simulink model "send_udp"  (R2016a)
settings: Solver=FixedStepAuto  StartTime=0.0  StopTime=inf  RelTol=1e-3
libraries: simulink_extras x4, etargetslib x2, instrumentlib x1
settings Model: Creator=Florian Wachter  LastModifiedBy=Florian Wachter

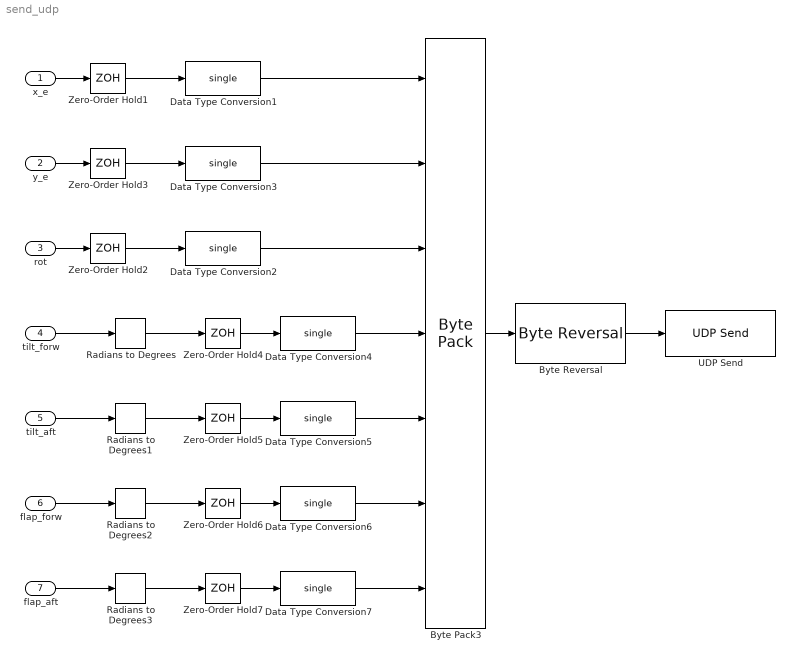
== system send_udp ==
  x_e : Inport
  y_e : Inport  Port=2
  rot : Inport  Port=3
  tilt_forw : Inport  Port=4
  tilt_aft : Inport  Port=5
  flap_forw : Inport  Port=6
  flap_aft : Inport  Port=7
  Byte Pack3 : etargetslib/Byte Pack  datatypes={'single','single','single','single','single','single','single'}  byteAlign=1
  Byte Reversal : etargetslib/Byte Reversal  numInp=1
  Data Type Conversion{1..7} (7 alike) : DataTypeConversion  OutDataTypeStr=single
  Radians to Degrees{,1..3} (4 alike) : simulink_extras/Transformations/Radians to Degrees
  UDP Send : instrumentlib/UDP Send  Host=localhost  Port=25000  LocalPort=-1  EnableBlockingMode=off  ByteOrder=BigEndian
  Zero-Order Hold{1..7} (7 alike) : ZeroOrderHold  SampleTime=1/30
  wires:
  tilt_forw/1 -> Radians to Degrees/1
  flap_forw/1 -> Radians to Degrees2/1
  Zero-Order Hold1/1 -> Data Type Conversion1/1
  Zero-Order Hold4/1 -> Data Type Conversion4/1
  Zero-Order Hold5/1 -> Data Type Conversion5/1
  Data Type Conversion5/1 -> Byte Pack3/5
  Data Type Conversion6/1 -> Byte Pack3/6
  Zero-Order Hold6/1 -> Data Type Conversion6/1
  Data Type Conversion4/1 -> Byte Pack3/4
  Data Type Conversion1/1 -> Byte Pack3/1
  x_e/1 -> Zero-Order Hold1/1
  Zero-Order Hold3/1 -> Data Type Conversion3/1
  y_e/1 -> Zero-Order Hold3/1
  tilt_aft/1 -> Radians to Degrees1/1
  Byte Reversal/1 -> UDP Send/1
  Byte Pack3/1 -> Byte Reversal/1
  Zero-Order Hold2/1 -> Data Type Conversion2/1
  rot/1 -> Zero-Order Hold2/1
  Data Type Conversion3/1 -> Byte Pack3/2
  Data Type Conversion2/1 -> Byte Pack3/3
  Radians to Degrees/1 -> Zero-Order Hold4/1
  Radians to Degrees1/1 -> Zero-Order Hold5/1
  Radians to Degrees2/1 -> Zero-Order Hold6/1
  flap_aft/1 -> Radians to Degrees3/1
  Data Type Conversion7/1 -> Byte Pack3/7
  Zero-Order Hold7/1 -> Data Type Conversion7/1
  Radians to Degrees3/1 -> Zero-Order Hold7/1
